simulink model "simulacao2a_works_but_height_is_160"  (R2020b)
settings: Solver=VariableStepAuto  StartTime=0.0  StopTime=100  FixedStep=0.0001
values from neighbouring files (symbols this model uses):
  b = 0.24    [droneINDI.m]
  B = 0.00029*[1 1 1 1]    [droneINDI.m]
  b_z = (8*KT(1)/m)*Omega_equilibrium    [droneINDI.m]
  delta_equilibrium = (Ke(1)*Omega(1) + R(1)*(KQ(1)*Omega(1) + B(1))*Omega(1)/Kt(1))/Vbat    [droneINDI.m]
  J = diag([3.8e-3,3.8e-3,7.1e-3])    [droneINDI.m]
  Jm = 1.4e-5*[1 1 1 1]    [droneINDI.m]
  Ke = 0.0247*[1 1 1 1]    [droneINDI.m]
  KQ = 1.2191e-5*[1 1 1 1]    [droneINDI.m]
  Kt = 0.0247*[1 1 1 1]    [droneINDI.m]
  KT = 3.5897e-5*[1 1 1 1]    [droneINDI.m]
  L = 0.00036*[1 1 1 1]    [droneINDI.m]
  m = 2    [droneINDI.m]
  Omega_equilibrium = sqrt(Force_each_motor/KT(1))    [droneINDI.m]
  R = 0.036*[1 1 1 1]    [droneINDI.m]
  Vbat = 15    [droneINDI.m]
undefined symbols (not defined in the file or in its folder): saturation
libraries: dspmtrx3 x19, vrlib x2, eeGeneralControl x1
settings Model: Creator=55159  LastModifiedBy=55159
settings DebuggingCC: UnderSpecifiedDimensionMsg=warning
settings HardwareCC: ProdHWDeviceType=AMD->x86-64 (Windows64)

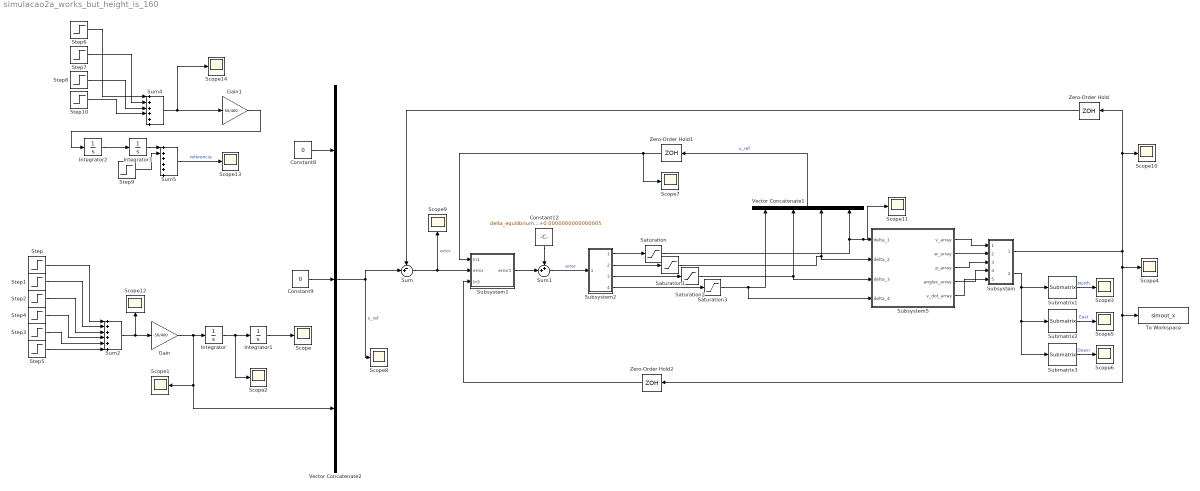
== system simulacao2a_works_but_height_is_160 ==
  Constant12 : Constant  Value=delta_equilibrium+0.0000000000000005
  Constant8 : Constant  Value=0
  Constant9 : Constant  Value=0
  Gain : Gain  Gain=-50/400
  Gain1 : Gain  Gain=-50/400
  Integrator{,1..3} (4 alike) : Integrator
  Saturation{,1..3} (4 alike) : Saturate  UpperLimit=saturation  LowerLimit=0
  Scope{,1..14} (15 alike) : Scope
  Step : Step  Time=30  SampleTime=0
  Step{1..2,7..8} (4 alike) : Step  Time=50  After=-1  SampleTime=0
  Step10 : Step  Time=70  SampleTime=0
  Step3 : Step  Time=0.5  After=-4*5  SampleTime=0
  Step4 : Step  Time=70  SampleTime=0
  Step5 : Step  Time=0.5+4.315  After=4*5  SampleTime=0
  Step6 : Step  Time=30  SampleTime=0
  Step9 : Step  Time=0.01  After=-18.3  SampleTime=0
  Submatrix1 : dspmtrx3/Submatrix  RowSpan=One row  RowStartMode=Index  RowStartIndex=1  RowEndMode=Last  RowEndIndex=1  ColSpan=One column  ColStartMode=First  ColStartIndex=1  ColEndMode=Last  ColEndIndex=1
  Submatrix2 : dspmtrx3/Submatrix  RowSpan=One row  RowStartMode=Index  RowStartIndex=2  RowEndMode=Last  RowEndIndex=1  ColSpan=One column  ColStartMode=First  ColStartIndex=1  ColEndMode=Last  ColEndIndex=1
  Submatrix3 : dspmtrx3/Submatrix  RowSpan=One row  RowStartMode=Index  RowStartIndex=3  RowEndMode=Last  RowEndIndex=1  ColSpan=One column  ColStartMode=First  ColStartIndex=1  ColEndMode=Last  ColEndIndex=1
  Subsystem : Subsystem
  Subsystem1 : Subsystem
  Subsystem2 : Subsystem
  Subsystem5 : Subsystem
  Sum : Sum  Inputs=-+|
  Sum1 : Sum  Inputs=++|
  Sum2 : Sum  Inputs=++++++
  Sum4 : Sum  Inputs=++++++
  Sum5 : Sum  Inputs=++++++
  To Workspace : ToWorkspace  VariableName=simout_x  SaveFormat=Timeseries  SampleTime=-1
  Vector Concatenate1 : Concatenate  NumInputs=4
  Vector Concatenate2 : Concatenate  NumInputs=3
  Zero-Order Hold : ZeroOrderHold  SampleTime=0.001
  Zero-Order Hold1 : ZeroOrderHold  SampleTime=0.001
  Zero-Order Hold2 : ZeroOrderHold  SampleTime=0.001
  wires:
  Vector Concatenate2/1 -> Sum/2, Scope8/1  "x_ref"
  Subsystem5/1(v_array) -> Subsystem/1(In1)
  Subsystem5/2(w_array) -> Subsystem/2(In2)
  Subsystem5/3(p_array) -> Subsystem/3(In3)
  Subsystem5/4(angles_array) -> Subsystem/4(In4)
  Subsystem/1(v_dot) -> Scope4/1, To Workspace/1, Zero-Order Hold2/1, Scope10/1, Zero-Order Hold/1
  Zero-Order Hold/1 -> Sum/1
  Subsystem2/3(Out3) -> Saturation2/1
  Subsystem2/2(Out2) -> Saturation1/1
  Subsystem2/4(Out4) -> Saturation3/1
  Subsystem2/1(Out1) -> Saturation/1
  Sum1/1 -> Subsystem2/1(In1)  "error"
  Vector Concatenate1/1 -> Zero-Order Hold1/1  "x_ref"
  Zero-Order Hold1/1 -> Scope7/1, Subsystem1/1(In1)
  Sum/1 -> Subsystem1/2(error), Scope9/1  "error"
  Zero-Order Hold2/1 -> Subsystem1/3(In3)
  Subsystem1/1(error1) -> Sum1/2
  Integrator1/1 -> Scope/1
  Gain/1 -> Vector Concatenate2/3, Scope1/1, Integrator/1
  Integrator/1 -> Scope2/1, Integrator1/1
  Step2/1 -> Sum2/3
  Step/1 -> Sum2/1
  Step1/1 -> Sum2/2
  Constant8/1 -> Vector Concatenate2/1
  Constant9/1 -> Vector Concatenate2/2
  Saturation/1 -> Vector Concatenate1/4, Scope11/1, Subsystem5/1(delta_1)
  Saturation1/1 -> Vector Concatenate1/3, Subsystem5/2(delta_2)
  Saturation2/1 -> Subsystem5/3(delta_3), Vector Concatenate1/2
  Saturation3/1 -> Vector Concatenate1/1, Subsystem5/4(delta_4)
  Subsystem/2(pos) -> Submatrix3/1, Submatrix2/1, Submatrix1/1
  Submatrix1/1 -> Scope3/1  "North"
  Submatrix2/1 -> Scope5/1  "East"
  Submatrix3/1 -> Scope6/1  "Down"
  Sum2/1 -> Gain/1, Scope12/1
  Constant12/1 -> Sum1/1
  Subsystem5/5(v_dot_array) -> Subsystem/5(v_dot_array)
  Step4/1 -> Sum2/4
  Step3/1 -> Sum2/5
  Step5/1 -> Sum2/6
  Sum4/1 -> Scope14/1, Gain1/1
  Integrator2/1 -> Integrator3/1
  Gain1/1 -> Integrator2/1
  Step7/1 -> Sum4/2
  Step10/1 -> Sum4/4
  Step8/1 -> Sum4/3
  Step6/1 -> Sum4/1
  Integrator3/1 -> Sum5/1
  Sum5/1 -> Scope13/1  "referencia"
  Step9/1 -> Sum5/2

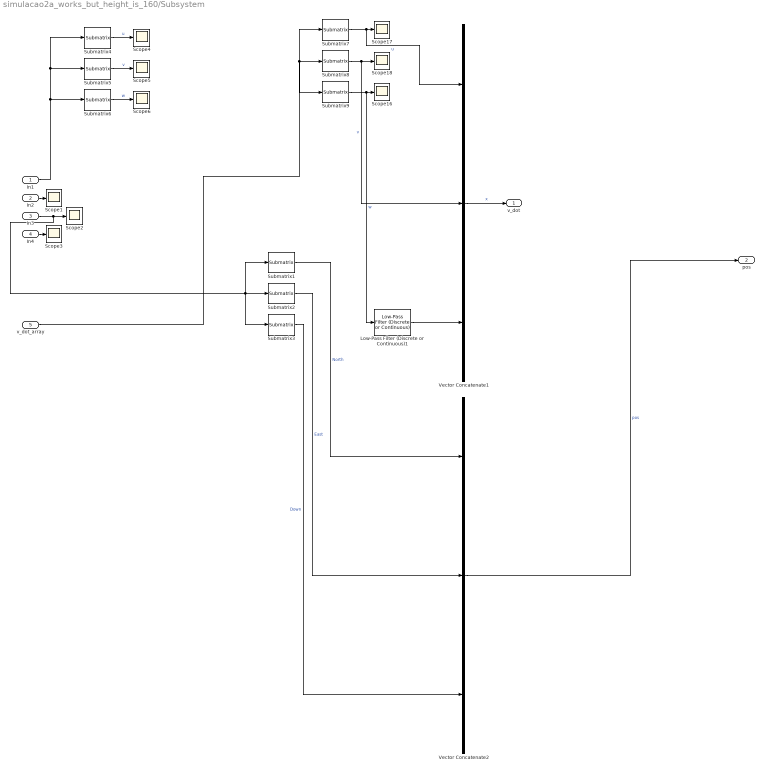
== system simulacao2a_works_but_height_is_160/Subsystem ==
  In1 : Inport
  In2 : Inport  Port=2
  In3 : Inport  Port=3
  In4 : Inport  Port=4
  v_dot_array : Inport  Port=5
  Low-Pass Filter (Discrete or Continuous)1 : eeGeneralControl/Low-Pass Filter (Discrete or Continuous)  K=1  T=1  B=inf  A=-inf  init_option=Inherited from block input  x0=0  Ts=-1
  Scope{1..6,16..18} (9 alike) : Scope
  Submatrix1 : dspmtrx3/Submatrix  RowSpan=One row  RowStartMode=Index  RowStartIndex=1  RowEndMode=Last  RowEndIndex=1  ColSpan=One column  ColStartMode=First  ColStartIndex=1  ColEndMode=Last  ColEndIndex=1
  Submatrix2 : dspmtrx3/Submatrix  RowSpan=One row  RowStartMode=Index  RowStartIndex=2  RowEndMode=Last  RowEndIndex=1  ColSpan=One column  ColStartMode=First  ColStartIndex=1  ColEndMode=Last  ColEndIndex=1
  Submatrix3 : dspmtrx3/Submatrix  RowSpan=One row  RowStartMode=Index  RowStartIndex=3  RowEndMode=Last  RowEndIndex=1  ColSpan=One column  ColStartMode=First  ColStartIndex=1  ColEndMode=Last  ColEndIndex=1
  Submatrix4 : dspmtrx3/Submatrix  RowSpan=One row  RowStartMode=Index  RowStartIndex=1  RowEndMode=Last  RowEndIndex=1  ColSpan=One column  ColStartMode=First  ColStartIndex=1  ColEndMode=Last  ColEndIndex=1
  Submatrix5 : dspmtrx3/Submatrix  RowSpan=One row  RowStartMode=Index  RowStartIndex=2  RowEndMode=Last  RowEndIndex=1  ColSpan=One column  ColStartMode=First  ColStartIndex=1  ColEndMode=Last  ColEndIndex=1
  Submatrix6 : dspmtrx3/Submatrix  RowSpan=One row  RowStartMode=Index  RowStartIndex=3  RowEndMode=Last  RowEndIndex=1  ColSpan=One column  ColStartMode=First  ColStartIndex=1  ColEndMode=Last  ColEndIndex=1
  Submatrix7 : dspmtrx3/Submatrix  RowSpan=One row  RowStartMode=Index  RowStartIndex=1  RowEndMode=Last  RowEndIndex=1  ColSpan=One column  ColStartMode=First  ColStartIndex=1  ColEndMode=Last  ColEndIndex=1
  Submatrix8 : dspmtrx3/Submatrix  RowSpan=One row  RowStartMode=Index  RowStartIndex=2  RowEndMode=Last  RowEndIndex=1  ColSpan=One column  ColStartMode=First  ColStartIndex=1  ColEndMode=Last  ColEndIndex=1
  Submatrix9 : dspmtrx3/Submatrix  RowSpan=One row  RowStartMode=Index  RowStartIndex=3  RowEndMode=Last  RowEndIndex=1  ColSpan=One column  ColStartMode=First  ColStartIndex=1  ColEndMode=Last  ColEndIndex=1
  Vector Concatenate1 : Concatenate  NumInputs=3
  Vector Concatenate2 : Concatenate  NumInputs=3
  v_dot : Outport  PortDimensions=[3 1]
  pos : Outport  Port=2  PortDimensions=[3 1]
  wires:
  Submatrix9/1 -> Low-Pass Filter (Discrete or Continuous)1/1, Scope16/1  "w"
  Submatrix8/1 -> Vector Concatenate1/2, Scope18/1  "v"
  Submatrix7/1 -> Vector Concatenate1/1, Scope17/1  "u"
  v_dot_array/1 -> Submatrix7/1, Submatrix9/1, Submatrix8/1
  Vector Concatenate1/1 -> v_dot/1  "x"
  In2/1 -> Scope1/1
  In4/1 -> Scope3/1
  In3/1 -> Submatrix1/1, Submatrix3/1, Submatrix2/1, Scope2/1
  Vector Concatenate2/1 -> pos/1  "pos"
  Submatrix1/1 -> Vector Concatenate2/1  "North"
  Submatrix2/1 -> Vector Concatenate2/2  "East"
  Submatrix3/1 -> Vector Concatenate2/3  "Down"
  Low-Pass Filter (Discrete or Continuous)1/1 -> Vector Concatenate1/3
  Submatrix6/1 -> Scope6/1  "w"
  In1/1 -> Submatrix5/1, Submatrix4/1, Submatrix6/1
  Submatrix4/1 -> Scope4/1  "u"
  Submatrix5/1 -> Scope5/1  "v"

== system simulacao2a_works_but_height_is_160/Subsystem1 ==
  In1 : Inport
  error : Inport  Port=2
  In3 : Inport  Port=3
  Gain : Gain  Gain=pinv([0 0 0 0; 0 0 0 0; -b_z -b_z -b_z -b_z])  Multiplication=Matrix(K*u) (u vector)
  Gain1 : Gain  Gain=1/(Omega_equilibrium/300)
  Scope{1..4,9} (5 alike) : Scope
  Sum2 : Sum  Inputs=+++
  error1 : Outport  PortDimensions=[4 1]
  wires:
  error/1 -> Scope9/1, Gain/1
  Sum2/1 -> Gain1/1  "error"
  Gain/1 -> Scope3/1, Sum2/2
  In1/1 -> Scope1/1
  In3/1 -> Scope2/1
  Gain1/1 -> Scope4/1, error1/1

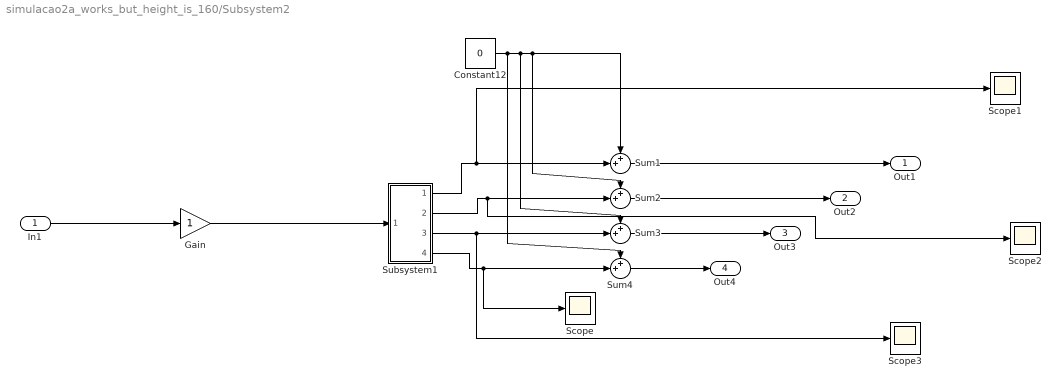
== system simulacao2a_works_but_height_is_160/Subsystem2 ==
  In1 : Inport
  Constant12 : Constant  Value=0
  Gain : Gain
  Scope{,1..3} (4 alike) : Scope
  Subsystem1 : Subsystem
  Sum{1..4} (4 alike) : Sum  Inputs=++|
  Out1 : Outport
  Out2 : Outport  Port=2
  Out3 : Outport  Port=3
  Out4 : Outport  Port=4
  wires:
  Subsystem1/2(Out2) -> Scope2/1, Sum2/2
  Subsystem1/1(Out1) -> Scope1/1, Sum1/2
  Constant12/1 -> Sum1/1, Sum2/1, Sum3/1, Sum4/1
  Sum4/1 -> Out4/1
  Subsystem1/3(Out3) -> Scope3/1, Sum3/2
  Subsystem1/4(Out4) -> Scope/1, Sum4/2
  Sum3/1 -> Out3/1
  Sum1/1 -> Out1/1
  Sum2/1 -> Out2/1
  In1/1 -> Gain/1
  Gain/1 -> Subsystem1/1(In1)

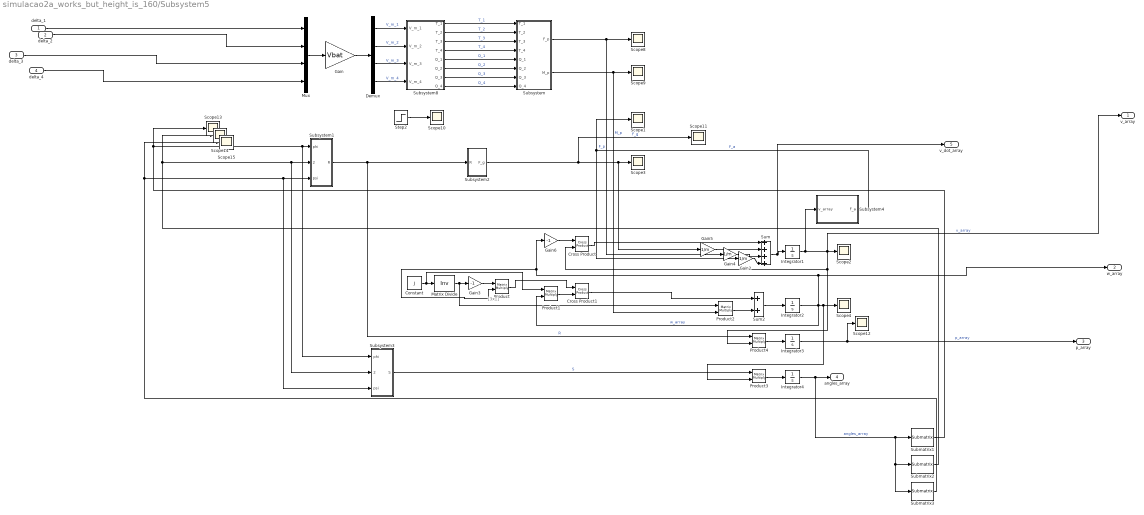
== system simulacao2a_works_but_height_is_160/Subsystem5 ==
  note: [3x1]
  delta_1 : Inport
  delta_2 : Inport  Port=2
  delta_3 : Inport  Port=3
  delta_4 : Inport  Port=4
  Constant : Constant  Value=J
  Cross Product : vrlib/Utilities/Cross Product
  Cross Product1 : vrlib/Utilities/Cross Product
  Demux : Demux
  Gain : Gain  Gain=Vbat
  Gain2 : Gain  Gain=1/m
  Gain3 : Gain  Gain=-1
  Gain4 : Gain  Gain=1/m
  Gain5 : Gain  Gain=1/m
  Gain6 : Gain  Gain=-1
  Integrator{1..4} (4 alike) : Integrator
  Matrix Divide : Product  Inputs=/  Multiplication=Matrix(*)
  Mux : Mux
  Product{,1..2,4} (4 alike) : Product  Multiplication=Matrix(*)
  Product3 : Product  Multiplication=Matrix(*)  InputSameDT=on
  Scope{1..4,8..15} (12 alike) : Scope
  Step2 : Step  SampleTime=0
  Submatrix1 : dspmtrx3/Submatrix  RowSpan=One row  RowStartMode=Index  RowStartIndex=1  RowEndMode=Last  RowEndIndex=1  ColSpan=One column  ColStartMode=First  ColStartIndex=1  ColEndMode=Last  ColEndIndex=1
  Submatrix2 : dspmtrx3/Submatrix  RowSpan=One row  RowStartMode=Index  RowStartIndex=2  RowEndMode=Last  RowEndIndex=1  ColSpan=One column  ColStartMode=Index  ColStartIndex=1  ColEndMode=Last  ColEndIndex=1
  Submatrix3 : dspmtrx3/Submatrix  RowSpan=One row  RowStartMode=Index  RowStartIndex=3  RowEndMode=Last  RowEndIndex=1  ColSpan=One column  ColStartMode=Index  ColStartIndex=1  ColEndMode=Last  ColEndIndex=1
  Subsystem : Subsystem
  Subsystem1 : Subsystem
  Subsystem2 : Subsystem
  Subsystem3 : Subsystem
  Subsystem4 : Subsystem
  Subsystem8 : Subsystem
  Sum : Sum  Inputs=++++
  Sum2 : Sum
  v_array : Outport
  w_array : Outport  Port=2
  p_array : Outport  Port=3
  angles_array : Outport  Port=4
  v_dot_array : Outport  Port=5
  wires:
  Subsystem8/7(Q_3) -> Subsystem/7(Q_3)  "Q_3"
  Sum/1 -> v_dot_array/1, Integrator1/1
  Integrator3/1 -> p_array/1, Scope12/1  "p_array"
  Subsystem/1(F_p) -> Scope8/1, Gain4/1  "F_p"
  Subsystem2/1(F_g) -> Scope11/1, Gain5/1, Scope3/1  "F_g"
  Subsystem4/1(F_a) -> Scope1/1, Gain2/1  "F_a"
  Integrator1/1 -> Subsystem4/1(v_array), v_array/1, Product4/2, Cross Product/2, Scope2/1  "v_array"
  Sum2/1 -> Integrator2/1
  Mux/1 -> Gain/1
  Gain/1 -> Demux/1
  Integrator2/1 -> Product1/2, w_array/1, Product/2, Gain6/1, Product3/2, Scope4/1  "w_array"
  Step2/1 -> Scope10/1
  Demux/3 -> Subsystem8/3(V_m_3)  "V_m_3"
  Subsystem1/1(R) -> Product4/1, Subsystem2/1(R)  "R"
  Gain2/1 -> Sum/4
  Submatrix3/1 -> Scope15/1, Subsystem3/3(psi), Subsystem1/3(psi)
  Subsystem8/1(T_1) -> Subsystem/1(T_1)  "T_1"
  Product4/1 -> Integrator3/1
  Subsystem3/1(S) -> Product3/1  "S"
  Product3/1 -> Integrator4/1
  Demux/1 -> Subsystem8/1(V_m_1)  "V_m_1"
  Demux/4 -> Subsystem8/4(V_m_4)  "V_m_4"
  Subsystem/2(M_p) -> Product2/2, Scope9/1  "M_p"
  Subsystem8/5(Q_1) -> Subsystem/5(Q_1)  "Q_1"
  Matrix Divide/1 -> Product2/1, Gain3/1
  Gain4/1 -> Sum/3
  Gain5/1 -> Sum/2
  Constant/1 -> Product1/1, Matrix Divide/1
  Gain3/1 -> Product/1
  Product1/1 -> Cross Product1/2
  Cross Product/1 -> Sum/1
  delta_3/1 -> Mux/3
  Gain6/1 -> Cross Product/1
  Submatrix2/1 -> Scope14/1, Subsystem3/2(theta), Subsystem1/2(theta)
  Subsystem8/2(T_2) -> Subsystem/2(T_2)  "T_2"
  Subsystem8/3(T_3) -> Subsystem/3(T_3)  "T_3"
  Subsystem8/4(T_4) -> Subsystem/4(T_4)  "T_4"
  Subsystem8/6(Q_2) -> Subsystem/6(Q_2)  "Q_2"
  Product/1 -> Cross Product1/1
  delta_4/1 -> Mux/4
  Subsystem8/8(Q_4) -> Subsystem/8(Q_4)  "Q_4"
  Demux/2 -> Subsystem8/2(V_m_2)  "V_m_2"
  Submatrix1/1 -> Scope13/1, Subsystem3/1(phi), Subsystem1/1(phi)
  Cross Product1/1 -> Sum2/1
  Product2/1 -> Sum2/2
  Integrator4/1 -> Submatrix3/1, Submatrix2/1, Submatrix1/1, angles_array/1  "angles_array"
  delta_1/1 -> Mux/1
  delta_2/1 -> Mux/2

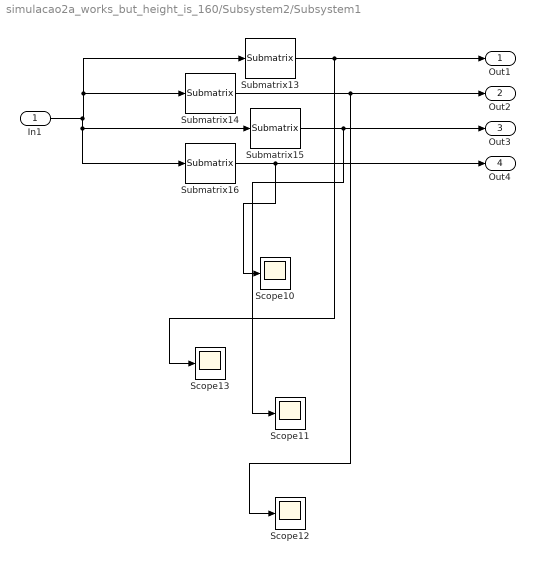
== system simulacao2a_works_but_height_is_160/Subsystem2/Subsystem1 ==
  In1 : Inport
  Scope{10..13} (4 alike) : Scope
  Submatrix13 : dspmtrx3/Submatrix  RowSpan=One row  RowStartMode=Index  RowStartIndex=1  RowEndMode=Last  RowEndIndex=1  ColSpan=One column  ColStartMode=First  ColStartIndex=1  ColEndMode=Last  ColEndIndex=1
  Submatrix14 : dspmtrx3/Submatrix  RowSpan=One row  RowStartMode=Index  RowStartIndex=2  RowEndMode=Last  RowEndIndex=1  ColSpan=One column  ColStartMode=Index  ColStartIndex=1  ColEndMode=Last  ColEndIndex=1
  Submatrix15 : dspmtrx3/Submatrix  RowSpan=One row  RowStartMode=Index  RowStartIndex=3  RowEndMode=Last  RowEndIndex=1  ColSpan=One column  ColStartMode=Index  ColStartIndex=1  ColEndMode=Last  ColEndIndex=1
  Submatrix16 : dspmtrx3/Submatrix  RowSpan=One row  RowStartMode=Index  RowStartIndex=4  RowEndMode=Last  RowEndIndex=1  ColSpan=One column  ColStartMode=Index  ColStartIndex=1  ColEndMode=Last  ColEndIndex=1
  Out1 : Outport
  Out2 : Outport  Port=2
  Out3 : Outport  Port=3
  Out4 : Outport  Port=4
  wires:
  In1/1 -> Submatrix16/1, Submatrix15/1, Submatrix13/1, Submatrix14/1
  Submatrix16/1 -> Out4/1, Scope10/1
  Submatrix14/1 -> Out2/1, Scope12/1
  Submatrix15/1 -> Out3/1, Scope11/1
  Submatrix13/1 -> Out1/1, Scope13/1

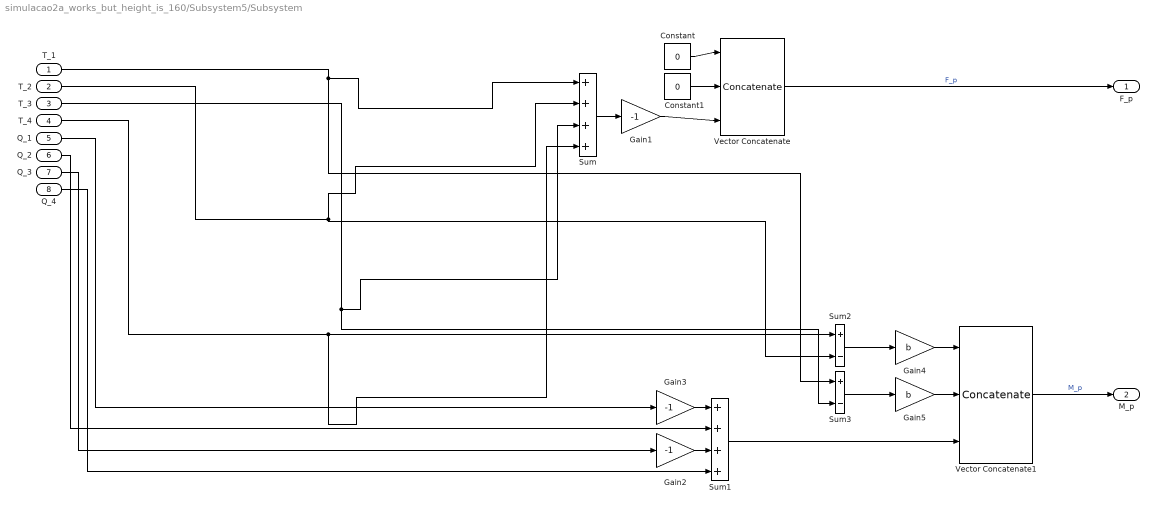
== system simulacao2a_works_but_height_is_160/Subsystem5/Subsystem ==
  T_1 : Inport
  T_2 : Inport  Port=2
  T_3 : Inport  Port=3
  T_4 : Inport  Port=4
  Q_1 : Inport  Port=5
  Q_2 : Inport  Port=6
  Q_3 : Inport  Port=7
  Q_4 : Inport  Port=8
  Constant : Constant  Value=0
  Constant1 : Constant  Value=0
  Gain1 : Gain  Gain=-1
  Gain2 : Gain  Gain=-1
  Gain3 : Gain  Gain=-1
  Gain4 : Gain  Gain=b
  Gain5 : Gain  Gain=b
  Sum : Sum  Inputs=++++
  Sum1 : Sum  Inputs=++++
  Sum2 : Sum  Inputs=+-
  Sum3 : Sum  Inputs=+-
  Vector Concatenate : Concatenate  NumInputs=3
  Vector Concatenate1 : Concatenate  NumInputs=3
  F_p : Outport  PortDimensions=[3 1]
  M_p : Outport  Port=2  PortDimensions=[3 1]
  wires:
  T_4/1 -> Sum/4, Sum2/1
  Q_1/1 -> Gain3/1
  Gain4/1 -> Vector Concatenate1/1
  T_3/1 -> Sum3/2, Sum/3
  T_1/1 -> Sum3/1, Sum/1
  Gain2/1 -> Sum1/3
  Constant1/1 -> Vector Concatenate/2
  Gain3/1 -> Sum1/1
  Sum2/1 -> Gain4/1
  Sum/1 -> Gain1/1
  Gain5/1 -> Vector Concatenate1/2
  Gain1/1 -> Vector Concatenate/3
  Constant/1 -> Vector Concatenate/1
  Vector Concatenate/1 -> F_p/1  "F_p"
  T_2/1 -> Sum/2, Sum2/2
  Sum1/1 -> Vector Concatenate1/3
  Sum3/1 -> Gain5/1
  Vector Concatenate1/1 -> M_p/1  "M_p"
  Q_2/1 -> Sum1/2
  Q_3/1 -> Gain2/1
  Q_4/1 -> Sum1/4

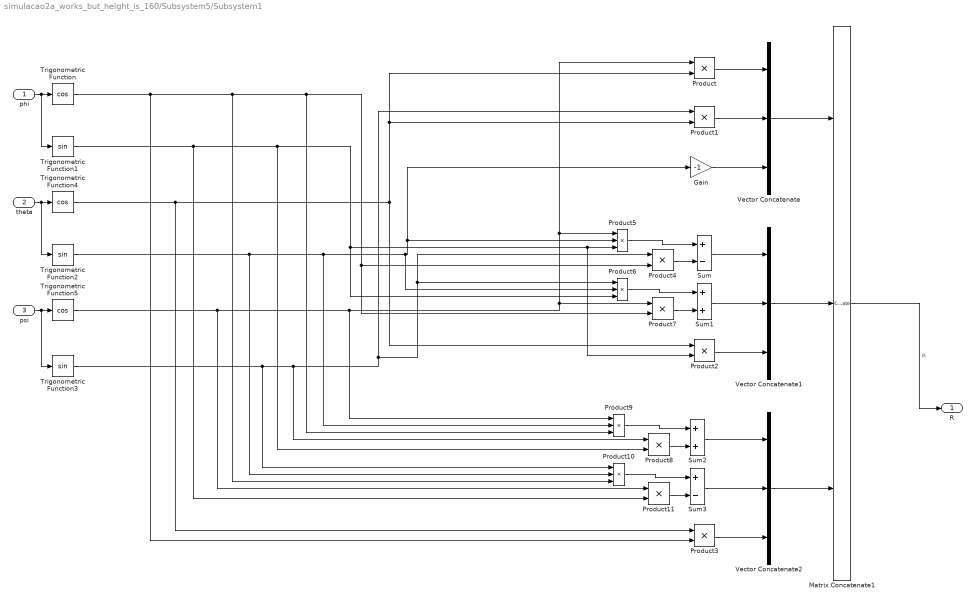
== system simulacao2a_works_but_height_is_160/Subsystem5/Subsystem1 ==
  phi : Inport
  theta : Inport  Port=2
  psi : Inport  Port=3
  Gain : Gain  Gain=-1
  Matrix Concatenate1 : Concatenate  NumInputs=3  Mode=Multidimensional array  ConcatenateDimension=2
  Product{,1..4,7..8,11} (8 alike) : Product
  Product{5..6,9..10} (4 alike) : Product  Inputs=3
  Sum : Sum  Inputs=+-
  Sum1 : Sum
  Sum2 : Sum
  Sum3 : Sum  Inputs=+-
  Trigonometric Function : Trigonometry  Operator=cos
  Trigonometric Function1 : Trigonometry
  Trigonometric Function2 : Trigonometry
  Trigonometric Function3 : Trigonometry
  Trigonometric Function4 : Trigonometry  Operator=cos
  Trigonometric Function5 : Trigonometry  Operator=cos
  Vector Concatenate : Concatenate  NumInputs=3  Mode=Multidimensional array
  Vector Concatenate1 : Concatenate  NumInputs=3  Mode=Multidimensional array
  Vector Concatenate2 : Concatenate  NumInputs=3  Mode=Multidimensional array
  R : Outport  PortDimensions=[3 3]
  wires:
  phi/1 -> Trigonometric Function1/1, Trigonometric Function/1
  theta/1 -> Trigonometric Function4/1, Trigonometric Function2/1
  psi/1 -> Trigonometric Function3/1, Trigonometric Function5/1
  Product/1 -> Vector Concatenate/1
  Product1/1 -> Vector Concatenate/2
  Sum1/1 -> Vector Concatenate1/2
  Sum/1 -> Vector Concatenate1/1
  Sum2/1 -> Vector Concatenate2/1
  Gain/1 -> Vector Concatenate/3
  Trigonometric Function5/1 -> Product11/1, Product9/1, Product7/1, Product5/1, Product/1
  Trigonometric Function4/1 -> Product3/1, Product1/2, Product/2, Product2/1
  Trigonometric Function3/1 -> Product10/1, Product8/1, Product6/1, Product4/1, Product1/1
  Product4/1 -> Sum/2
  Product5/1 -> Sum/1
  Trigonometric Function2/1 -> Product10/2, Product9/2, Product6/2, Gain/1, Product5/2
  Trigonometric Function1/1 -> Product11/2, Product8/2, Product6/3, Product5/3, Product2/2
  Trigonometric Function/1 -> Product3/2, Product10/3, Product9/3, Product7/2, Product4/2
  Product6/1 -> Sum1/1
  Product7/1 -> Sum1/2
  Product2/1 -> Vector Concatenate1/3
  Product9/1 -> Sum2/1
  Product10/1 -> Sum3/1
  Product8/1 -> Sum2/2
  Product11/1 -> Sum3/2
  Product3/1 -> Vector Concatenate2/3
  Vector Concatenate/1 -> Matrix Concatenate1/1
  Vector Concatenate1/1 -> Matrix Concatenate1/2
  Vector Concatenate2/1 -> Matrix Concatenate1/3
  Matrix Concatenate1/1 -> R/1  "R"
  Sum3/1 -> Vector Concatenate2/2

== system simulacao2a_works_but_height_is_160/Subsystem5/Subsystem2 ==
  R : Inport
  Constant : Constant  Value=0
  Constant1 : Constant  Value=0
  Gain2 : Gain  Gain=m
  Product : Product  Multiplication=Matrix(*)
  Step : Step  Time=0  After=9.81  SampleTime=0
  Transpose : Math  Operator=transpose  SaturateOnIntegerOverflow=on
  Vector Concatenate : Concatenate  NumInputs=3
  F_g : Outport
  wires:
  Constant/1 -> Vector Concatenate/1
  R/1 -> Transpose/1
  Gain2/1 -> Product/1
  Constant1/1 -> Vector Concatenate/2
  Vector Concatenate/1 -> Product/2
  Product/1 -> F_g/1  "F_g"
  Transpose/1 -> Gain2/1
  Step/1 -> Vector Concatenate/3

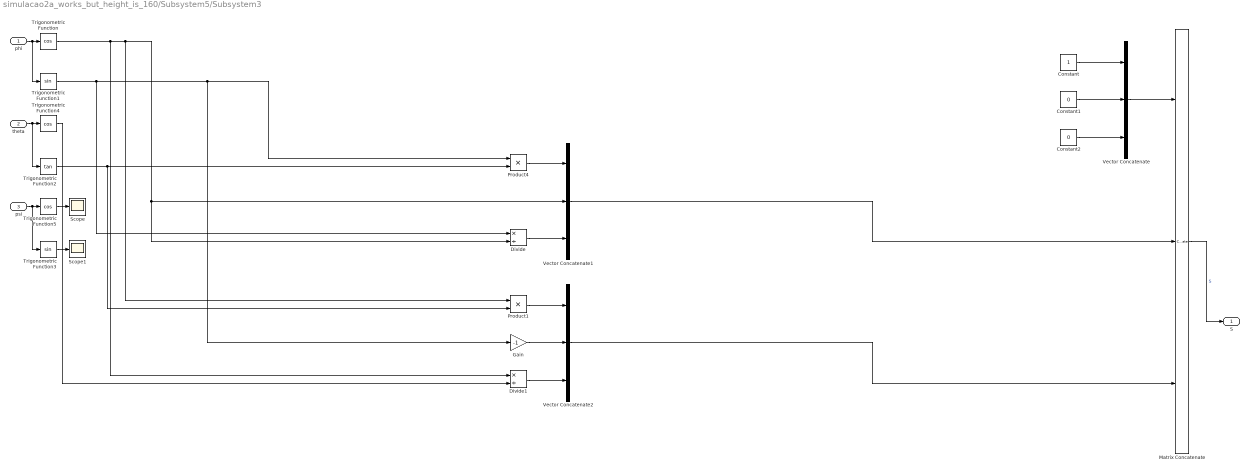
== system simulacao2a_works_but_height_is_160/Subsystem5/Subsystem3 ==
  phi : Inport
  theta : Inport  Port=2
  psi : Inport  Port=3
  Constant : Constant
  Constant1 : Constant  Value=0
  Constant2 : Constant  Value=0
  Divide : Product  Inputs=*/
  Divide1 : Product  Inputs=*/
  Gain : Gain  Gain=-1
  Matrix Concatenate : Concatenate  NumInputs=3  Mode=Multidimensional array  ConcatenateDimension=2
  Product1 : Product
  Product4 : Product
  Scope : Scope
  Scope1 : Scope
  Trigonometric Function : Trigonometry  Operator=cos
  Trigonometric Function1 : Trigonometry
  Trigonometric Function2 : Trigonometry  Operator=tan
  Trigonometric Function3 : Trigonometry
  Trigonometric Function4 : Trigonometry  Operator=cos
  Trigonometric Function5 : Trigonometry  Operator=cos
  Vector Concatenate : Concatenate  NumInputs=3
  Vector Concatenate1 : Concatenate  NumInputs=3
  Vector Concatenate2 : Concatenate  NumInputs=3
  S : Outport  PortDimensions=[3 3]
  wires:
  Matrix Concatenate/1 -> S/1  "S"
  phi/1 -> Trigonometric Function1/1, Trigonometric Function/1
  theta/1 -> Trigonometric Function4/1, Trigonometric Function2/1
  psi/1 -> Trigonometric Function3/1, Trigonometric Function5/1
  Divide/1 -> Vector Concatenate1/3
  Constant/1 -> Vector Concatenate/1
  Constant1/1 -> Vector Concatenate/2
  Constant2/1 -> Vector Concatenate/3
  Trigonometric Function/1 -> Divide1/1, Product1/1, Divide/2, Vector Concatenate1/2
  Product4/1 -> Vector Concatenate1/1
  Divide1/1 -> Vector Concatenate2/3
  Gain/1 -> Vector Concatenate2/2
  Product1/1 -> Vector Concatenate2/1
  Trigonometric Function1/1 -> Divide/1, Gain/1, Product4/1
  Trigonometric Function2/1 -> Product1/2, Product4/2
  Trigonometric Function4/1 -> Divide1/2
  Trigonometric Function5/1 -> Scope/1
  Trigonometric Function3/1 -> Scope1/1
  Vector Concatenate/1 -> Matrix Concatenate/1
  Vector Concatenate1/1 -> Matrix Concatenate/2
  Vector Concatenate2/1 -> Matrix Concatenate/3

== system simulacao2a_works_but_height_is_160/Subsystem5/Subsystem4 ==
  v_array : Inport
  Dot Product : DotProduct  InputSameDT=on  OutDataTypeStr=Inherit: Inherit via internal rule
  Gain7 : Gain  Gain=-0.254274793/10
  Product5 : Product
  Scope : Scope
  Sqrt : Sqrt  SaturateOnIntegerOverflow=on
  F_a : Outport  PortDimensions=[3 1]
  wires:
  v_array/1 -> Dot Product/2, Product5/1, Dot Product/1
  Product5/1 -> Gain7/1
  Sqrt/1 -> Product5/2
  Dot Product/1 -> Sqrt/1
  Gain7/1 -> Scope/1, F_a/1  "F_a"

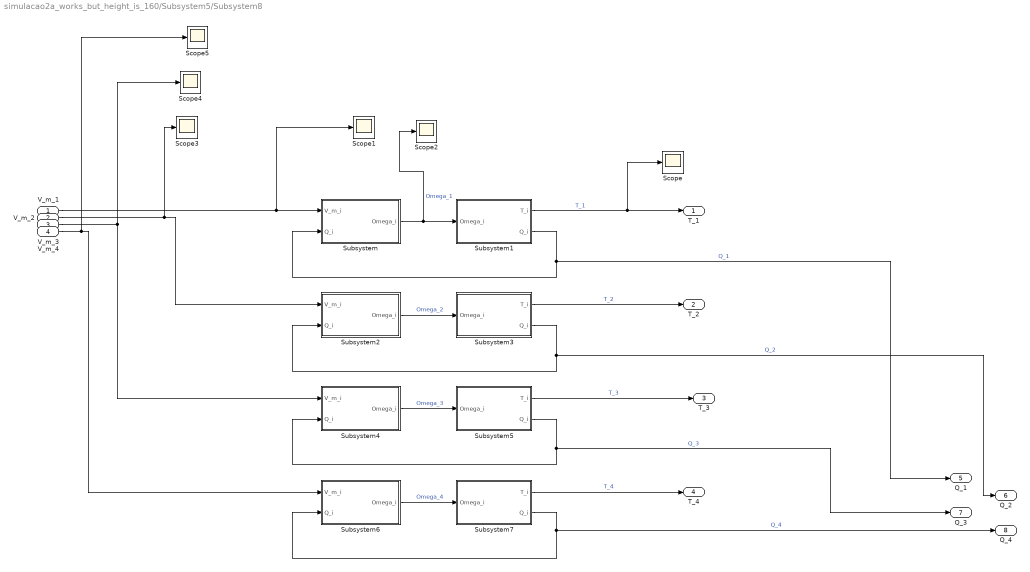
== system simulacao2a_works_but_height_is_160/Subsystem5/Subsystem8 ==
  V_m_1 : Inport
  V_m_2 : Inport  Port=2
  V_m_3 : Inport  Port=3
  V_m_4 : Inport  Port=4
  Scope{,1..5} (6 alike) : Scope
  Subsystem : Subsystem
  Subsystem1 : Subsystem
  Subsystem2 : Subsystem
  Subsystem3 : Subsystem
  Subsystem4 : Subsystem
  Subsystem5 : Subsystem
  Subsystem6 : Subsystem
  Subsystem7 : Subsystem
  T_1 : Outport
  T_2 : Outport  Port=2
  T_3 : Outport  Port=3
  T_4 : Outport  Port=4
  Q_1 : Outport  Port=5
  Q_2 : Outport  Port=6
  Q_3 : Outport  Port=7
  Q_4 : Outport  Port=8
  wires:
  Subsystem6/1(Omega_i) -> Subsystem7/1(Omega_i)  "Omega_4"
  Subsystem3/2(Q_i) -> Q_2/1, Subsystem2/2(Q_i)  "Q_2"
  Subsystem7/2(Q_i) -> Subsystem6/2(Q_i), Q_4/1  "Q_4"
  Subsystem1/2(Q_i) -> Q_1/1, Subsystem/2(Q_i)  "Q_1"
  Subsystem/1(Omega_i) -> Scope2/1, Subsystem1/1(Omega_i)  "Omega_1"
  V_m_1/1 -> Scope1/1, Subsystem/1(V_m_i)
  V_m_2/1 -> Scope3/1, Subsystem2/1(V_m_i)
  Subsystem1/1(T_i) -> Scope/1, T_1/1  "T_1"
  Subsystem5/2(Q_i) -> Q_3/1, Subsystem4/2(Q_i)  "Q_3"
  Subsystem4/1(Omega_i) -> Subsystem5/1(Omega_i)  "Omega_3"
  Subsystem2/1(Omega_i) -> Subsystem3/1(Omega_i)  "Omega_2"
  Subsystem7/1(T_i) -> T_4/1  "T_4"
  Subsystem5/1(T_i) -> T_3/1  "T_3"
  Subsystem3/1(T_i) -> T_2/1  "T_2"
  V_m_4/1 -> Scope5/1, Subsystem6/1(V_m_i)
  V_m_3/1 -> Subsystem4/1(V_m_i), Scope4/1

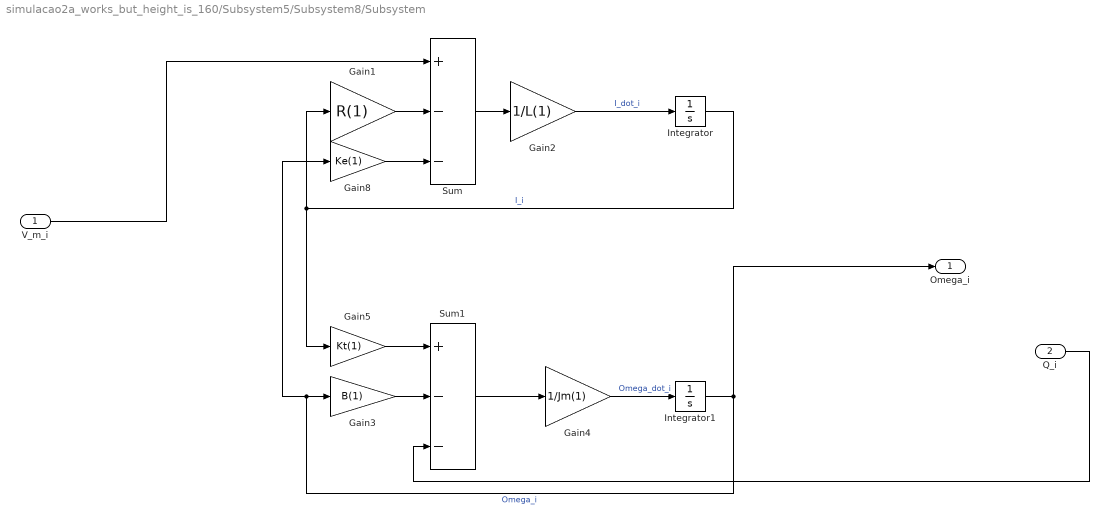
== system simulacao2a_works_but_height_is_160/Subsystem5/Subsystem8/Subsystem ==
  V_m_i : Inport
  Q_i : Inport  Port=2
  Gain1 : Gain  Gain=R(1)
  Gain2 : Gain  Gain=1/L(1)
  Gain3 : Gain  Gain=B(1)
  Gain4 : Gain  Gain=1/Jm(1)
  Gain5 : Gain  Gain=Kt(1)
  Gain8 : Gain  Gain=Ke(1)
  Integrator : Integrator
  Integrator1 : Integrator
  Sum : Sum  Inputs=+--
  Sum1 : Sum  Inputs=+--
  Omega_i : Outport
  wires:
  Gain4/1 -> Integrator1/1  "Omega_dot_i"
  V_m_i/1 -> Sum/1
  Integrator1/1 -> Omega_i/1, Gain8/1, Gain3/1  "Omega_i"
  Sum/1 -> Gain2/1
  Q_i/1 -> Sum1/3
  Sum1/1 -> Gain4/1
  Gain1/1 -> Sum/2
  Gain8/1 -> Sum/3
  Integrator/1 -> Gain1/1, Gain5/1  "I_i"
  Gain5/1 -> Sum1/1
  Gain3/1 -> Sum1/2
  Gain2/1 -> Integrator/1  "I_dot_i"

== system simulacao2a_works_but_height_is_160/Subsystem5/Subsystem8/Subsystem1 ==
  Omega_i : Inport
  Gain6 : Gain  Gain=KT(1)
  Gain7 : Gain  Gain=KQ(1)
  Math Function : Math  Operator=square  SaturateOnIntegerOverflow=on
  T_i : Outport
  Q_i : Outport  Port=2
  wires:
  Gain6/1 -> T_i/1  "T_i"
  Math Function/1 -> Gain7/1, Gain6/1
  Omega_i/1 -> Math Function/1
  Gain7/1 -> Q_i/1  "Q_i"

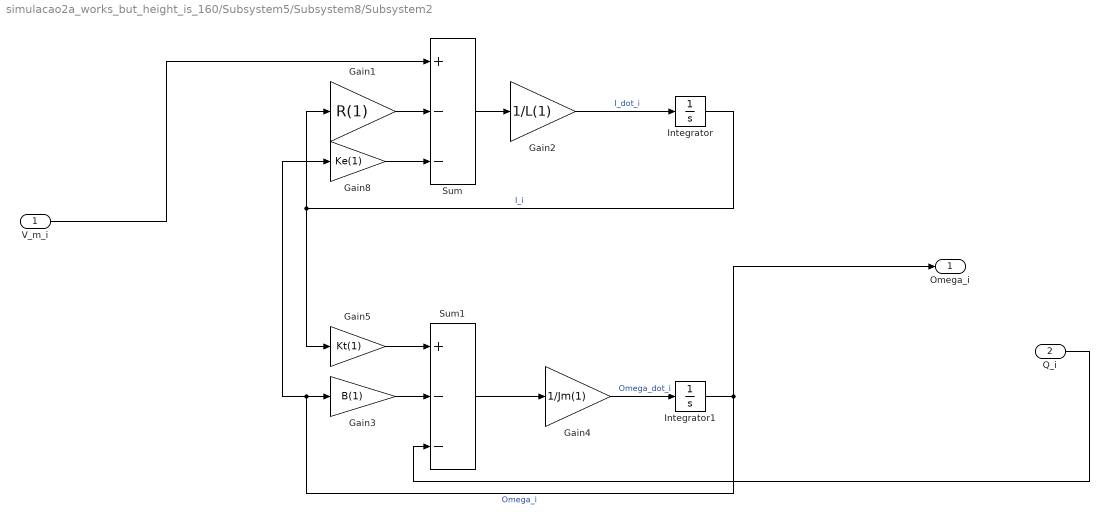
== system simulacao2a_works_but_height_is_160/Subsystem5/Subsystem8/Subsystem2 ==
  V_m_i : Inport
  Q_i : Inport  Port=2
  Gain1 : Gain  Gain=R(1)
  Gain2 : Gain  Gain=1/L(1)
  Gain3 : Gain  Gain=B(1)
  Gain4 : Gain  Gain=1/Jm(1)
  Gain5 : Gain  Gain=Kt(1)
  Gain8 : Gain  Gain=Ke(1)
  Integrator : Integrator
  Integrator1 : Integrator
  Sum : Sum  Inputs=+--
  Sum1 : Sum  Inputs=+--
  Omega_i : Outport
  wires:
  Gain4/1 -> Integrator1/1  "Omega_dot_i"
  V_m_i/1 -> Sum/1
  Integrator1/1 -> Omega_i/1, Gain8/1, Gain3/1  "Omega_i"
  Sum/1 -> Gain2/1
  Q_i/1 -> Sum1/3
  Sum1/1 -> Gain4/1
  Gain1/1 -> Sum/2
  Gain8/1 -> Sum/3
  Integrator/1 -> Gain1/1, Gain5/1  "I_i"
  Gain5/1 -> Sum1/1
  Gain3/1 -> Sum1/2
  Gain2/1 -> Integrator/1  "I_dot_i"

== system simulacao2a_works_but_height_is_160/Subsystem5/Subsystem8/Subsystem3 ==
  Omega_i : Inport
  Gain6 : Gain  Gain=KT(1)
  Gain7 : Gain  Gain=KQ(1)
  Math Function : Math  Operator=square  SaturateOnIntegerOverflow=on
  T_i : Outport
  Q_i : Outport  Port=2
  wires:
  Gain6/1 -> T_i/1  "T_i"
  Math Function/1 -> Gain7/1, Gain6/1
  Omega_i/1 -> Math Function/1
  Gain7/1 -> Q_i/1  "Q_i"

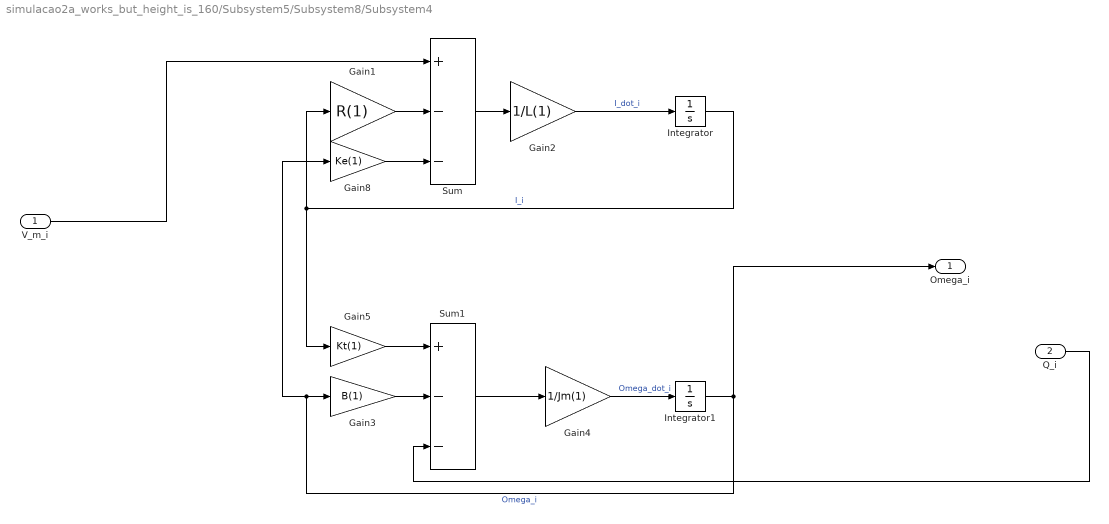
== system simulacao2a_works_but_height_is_160/Subsystem5/Subsystem8/Subsystem4 ==
  V_m_i : Inport
  Q_i : Inport  Port=2
  Gain1 : Gain  Gain=R(1)
  Gain2 : Gain  Gain=1/L(1)
  Gain3 : Gain  Gain=B(1)
  Gain4 : Gain  Gain=1/Jm(1)
  Gain5 : Gain  Gain=Kt(1)
  Gain8 : Gain  Gain=Ke(1)
  Integrator : Integrator
  Integrator1 : Integrator
  Sum : Sum  Inputs=+--
  Sum1 : Sum  Inputs=+--
  Omega_i : Outport
  wires:
  Gain4/1 -> Integrator1/1  "Omega_dot_i"
  V_m_i/1 -> Sum/1
  Integrator1/1 -> Omega_i/1, Gain8/1, Gain3/1  "Omega_i"
  Sum/1 -> Gain2/1
  Q_i/1 -> Sum1/3
  Sum1/1 -> Gain4/1
  Gain1/1 -> Sum/2
  Gain8/1 -> Sum/3
  Integrator/1 -> Gain1/1, Gain5/1  "I_i"
  Gain5/1 -> Sum1/1
  Gain3/1 -> Sum1/2
  Gain2/1 -> Integrator/1  "I_dot_i"

== system simulacao2a_works_but_height_is_160/Subsystem5/Subsystem8/Subsystem5 ==
  Omega_i : Inport
  Gain6 : Gain  Gain=KT(1)
  Gain7 : Gain  Gain=KQ(1)
  Math Function : Math  Operator=square  SaturateOnIntegerOverflow=on
  T_i : Outport
  Q_i : Outport  Port=2
  wires:
  Gain6/1 -> T_i/1  "T_i"
  Math Function/1 -> Gain7/1, Gain6/1
  Omega_i/1 -> Math Function/1
  Gain7/1 -> Q_i/1  "Q_i"

== system simulacao2a_works_but_height_is_160/Subsystem5/Subsystem8/Subsystem6 ==
  V_m_i : Inport
  Q_i : Inport  Port=2
  Gain1 : Gain  Gain=R(1)
  Gain2 : Gain  Gain=1/L(1)
  Gain3 : Gain  Gain=B(1)
  Gain4 : Gain  Gain=1/Jm(1)
  Gain5 : Gain  Gain=Kt(1)
  Gain8 : Gain  Gain=Ke(1)
  Integrator : Integrator
  Integrator1 : Integrator
  Sum : Sum  Inputs=+--
  Sum1 : Sum  Inputs=+--
  Omega_i : Outport
  wires:
  Gain4/1 -> Integrator1/1  "Omega_dot_i"
  V_m_i/1 -> Sum/1
  Integrator1/1 -> Omega_i/1, Gain8/1, Gain3/1  "Omega_i"
  Sum/1 -> Gain2/1
  Q_i/1 -> Sum1/3
  Sum1/1 -> Gain4/1
  Gain1/1 -> Sum/2
  Gain8/1 -> Sum/3
  Integrator/1 -> Gain1/1, Gain5/1  "I_i"
  Gain5/1 -> Sum1/1
  Gain3/1 -> Sum1/2
  Gain2/1 -> Integrator/1  "I_dot_i"

== system simulacao2a_works_but_height_is_160/Subsystem5/Subsystem8/Subsystem7 ==
  Omega_i : Inport
  Gain6 : Gain  Gain=KT(1)
  Gain7 : Gain  Gain=KQ(1)
  Math Function : Math  Operator=square  SaturateOnIntegerOverflow=on
  T_i : Outport
  Q_i : Outport  Port=2
  wires:
  Gain6/1 -> T_i/1  "T_i"
  Math Function/1 -> Gain7/1, Gain6/1
  Omega_i/1 -> Math Function/1
  Gain7/1 -> Q_i/1  "Q_i"
